simulink model "proj2sim"  (R2024b)
settings: Solver=VariableStepAuto  StartTime=0.0  StopTime=10.0  RelTol=1e-3
values from neighbouring files (symbols this model uses):
  F = inv(C*inv(-A+B*K)*B)    [proj2.m]
  K = place(A, B, desiredPoles)    [proj2.m]
  L = place(A', C', desiredObserverPoles)'    [proj2.m]
undefined symbols (not defined in the file or in its folder): A, B, C
settings Model: Creator=steve0gillet  LastModifiedBy=steve0gillet

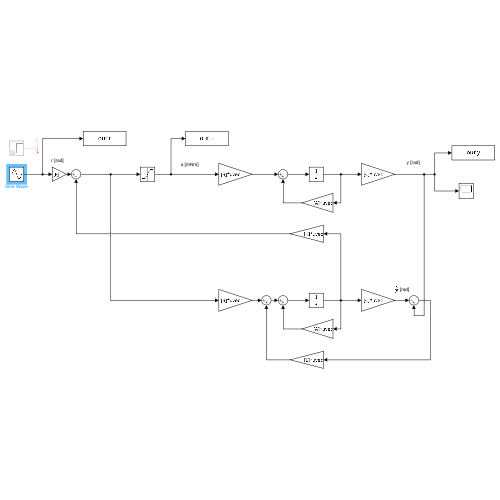
[thumbnail: Simulink's stored preview of the top-level diagram]
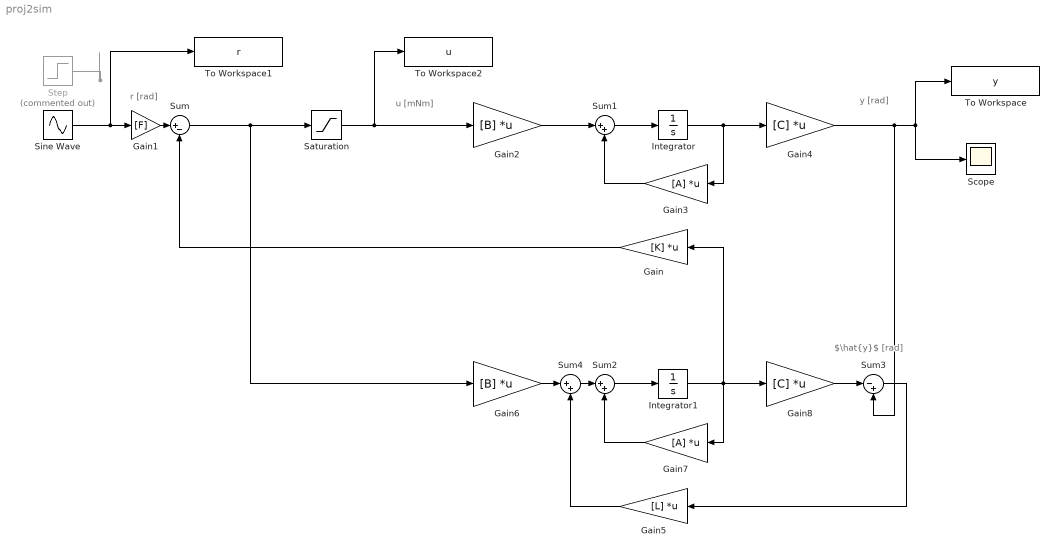
== system proj2sim ==
  note: y [rad]
  note: r [rad]
  note: u [mNm]
  note: $\hat{y}$ [rad]
  Gain : Gain  Gain=[K]  Multiplication=Matrix(K*u) (u vector)
  Gain1 : Gain  Gain=[F]
  Gain2 : Gain  Gain=[B]  Multiplication=Matrix(K*u) (u vector)
  Gain3 : Gain  Gain=[A]  Multiplication=Matrix(K*u) (u vector)
  Gain4 : Gain  Gain=[C]  Multiplication=Matrix(K*u) (u vector)
  Gain5 : Gain  Gain=[L]  Multiplication=Matrix(K*u) (u vector)
  Gain6 : Gain  Gain=[B]  Multiplication=Matrix(K*u) (u vector)
  Gain7 : Gain  Gain=[A]  Multiplication=Matrix(K*u) (u vector)
  Gain8 : Gain  Gain=[C]  Multiplication=Matrix(K*u) (u vector)
  Integrator : Integrator
  Integrator1 : Integrator
  Saturation : Saturate  UpperLimit=67  LowerLimit=-67
  Scope : Scope
  Sine Wave : Sin  Amplitude=0.1  Frequency=1*2*pi  SampleTime=0
  Step : Step  Commented=on  After=0.1  SampleTime=0
  Sum : Sum  Inputs=|+-
  Sum1 : Sum  Inputs=|++
  Sum2 : Sum  Inputs=|++
  Sum3 : Sum  Inputs=|-+
  Sum4 : Sum  Inputs=|++
  To Workspace : ToWorkspace  VariableName=y  SaveFormat=Timeseries  SampleTime=-1
  To Workspace1 : ToWorkspace  VariableName=r  SaveFormat=Timeseries  SampleTime=-1
  To Workspace2 : ToWorkspace  VariableName=u  SaveFormat=Timeseries  SampleTime=-1
  wires:
  Saturation/1 -> To Workspace2/1, Gain2/1
  Step/1 -> ?
  Sum/1 -> Gain6/1, Saturation/1
  Gain4/1 -> Scope/1, To Workspace/1, Sum3/2
  Gain/1 -> Sum/2
  Gain1/1 -> Sum/1
  Gain2/1 -> Sum1/1
  Sum1/1 -> Integrator/1
  Integrator/1 -> Gain3/1, Gain4/1
  Gain3/1 -> Sum1/2
  Sine Wave/1 -> To Workspace1/1, Gain1/1
  Sum2/1 -> Integrator1/1
  Integrator1/1 -> Gain/1, Gain7/1, Gain8/1
  Gain7/1 -> Sum2/2
  Gain8/1 -> Sum3/1
  Sum3/1 -> Gain5/1
  Gain6/1 -> Sum4/1
  Sum4/1 -> Sum2/1
  Gain5/1 -> Sum4/2
